simulink model "SineWave1"  (R2017b)
settings: Solver=FixedStepDiscrete  StartTime=0.0  StopTime=10.0  FixedStep=1.000000  RelTol=1e-3
settings Model: Creator=hbourbou  LastModifiedBy=hbourbou

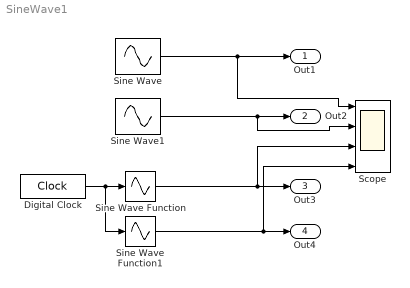
== system SineWave1 ==
  Digital Clock : DigitalClock
  Scope : Scope  NumInputPorts=4
  Sine Wave : Sin  SampleTime=0
  Sine Wave Function : Sin  SineType=Sample based  TimeSource=Use external signal  SampleTime=0
  Sine Wave Function1 : Sin  TimeSource=Use external signal  SampleTime=0
  Sine Wave1 : Sin  SineType=Sample based  SampleTime=1
  Out1 : Outport
  Out2 : Outport  Port=2
  Out3 : Outport  Port=3
  Out4 : Outport  Port=4
  wires:
  Sine Wave/1 -> Scope/1, Out1/1
  Digital Clock/1 -> Sine Wave Function1/1, Sine Wave Function/1
  Sine Wave1/1 -> Scope/2, Out2/1
  Sine Wave Function/1 -> Scope/3, Out3/1
  Sine Wave Function1/1 -> Scope/4, Out4/1
